simulink model "Task_1_24_Model"  (R2024b)
settings: Solver=VariableStepAuto  StartTime=0.0  StopTime=10.0  RelTol=1e-3
settings Model: Creator=omari  LastModifiedBy=omari

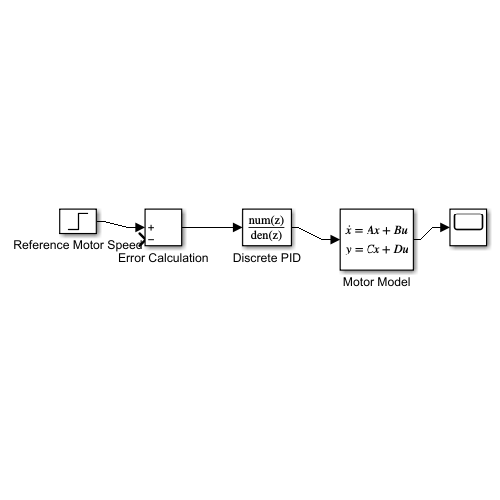
[thumbnail: Simulink's stored preview of the top-level diagram]
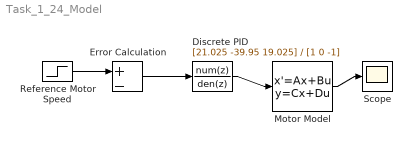
== system Task_1_24_Model ==
  Discrete PID : DiscreteTransferFcn  Numerator=[21.025 -39.95 19.025]  Denominator=[1 0 -1]  SampleTime=0.01
  Error Calculation : Sum  Inputs=|+-
  Motor Model : StateSpace  A=-0.5  D=0  InitialCondition=0
  Reference Motor Speed : Step  SampleTime=0
  Scope : Scope
  wires:
  Reference Motor Speed/1 -> Error Calculation/1
  Error Calculation/1 -> Discrete PID/1
  Discrete PID/1 -> Motor Model/1
  Motor Model/1 -> Scope/1
